simulink model "structuri_avansate"  (R2024a)
settings: Solver=VariableStepAuto  StartTime=0.0  StopTime=1000  RelTol=1e-3
values from neighbouring files (symbols this model uses):
  C = 9    [Proiect.m]
  h0 = 16.78    [Proiect.m]
  h1 = 19.66    [Proiect.m]
  k = 0.035    [Proiect.m]
  k11 = k2*k2+4*(k-k3)*k1    (= 0.0890826)    [Proiect.m]
  k12 = 8*(k-k3)    (= 0.2848)    [Proiect.m]
  k13 = 2*(k-k3)    (= 0.0712)    [Proiect.m]
  k2 = -0.015    [Proiect.m]
  kcompensare = (delta_h/(q1-q0))/(delta_h/delta_ua)    (= 0.16393442623)    [Proiect.m]
  kp = (delta_h/3)/delta_ua    (= 1.92)    [Proiect.m]
  q0 = 37.07    [Proiect.m]
undefined symbols (not defined in the file or in its folder): ki, ki1, ki2, kp1, kp2
libraries: slpidlib x6
(part 2 of 2)

== system structuri_avansate/ModelProces 3/Pompa/k11  ==
  k : Inport
  Add : Sum
  Constant : Constant  Value=4
  Product : Product
  Product1 : Product  Inputs=3
  Subtract : Sum  Inputs=+-
  k1 : Constant  Value=0.624
  k2 : Constant  Value=-0.015
  k3 : Constant  Value=-0.0006
  k11 : Outport
  wires:
  k2/1 -> Product/2, Product/1
  k/1 -> Subtract/1
  k3/1 -> Subtract/2
  Subtract/1 -> Product1/1
  k1/1 -> Product1/2
  Constant/1 -> Product1/3
  Product1/1 -> Add/1
  Product/1 -> Add/2
  Add/1 -> k11/1

== system structuri_avansate/ModelProces 3/Pompa/k12 ==
  k : Inport
  Product1 : Product
  Subtract : Sum  Inputs=+-
  "constant " : Constant  Value=8
  k3 : Constant  Value=-0.0006
  k12 : Outport
  wires:
  k/1 -> Subtract/1
  k3/1 -> Subtract/2
  Subtract/1 -> Product1/1
  "constant "/1 -> Product1/2
  Product1/1 -> k12/1

== system structuri_avansate/ModelProces 3/Pompa/k13 ==
  k : Inport
  Product1 : Product
  Subtract : Sum  Inputs=+-
  "constant " : Constant  Value=2
  k3 : Constant  Value=-0.0006
  k13 : Outport
  wires:
  k/1 -> Subtract/1
  k3/1 -> Subtract/2
  Subtract/1 -> Product1/1
  "constant "/1 -> Product1/2
  Product1/1 -> k13/1

== system structuri_avansate/ModelProces 4/Pompa/k11  ==
  k : Inport
  Add : Sum
  Constant : Constant  Value=4
  Product : Product
  Product1 : Product  Inputs=3
  Subtract : Sum  Inputs=+-
  k1 : Constant  Value=0.624
  k2 : Constant  Value=-0.015
  k3 : Constant  Value=-0.0006
  k11 : Outport
  wires:
  k2/1 -> Product/2, Product/1
  k/1 -> Subtract/1
  k3/1 -> Subtract/2
  Subtract/1 -> Product1/1
  k1/1 -> Product1/2
  Constant/1 -> Product1/3
  Product1/1 -> Add/1
  Product/1 -> Add/2
  Add/1 -> k11/1

== system structuri_avansate/ModelProces 4/Pompa/k12 ==
  k : Inport
  Product1 : Product
  Subtract : Sum  Inputs=+-
  "constant " : Constant  Value=8
  k3 : Constant  Value=-0.0006
  k12 : Outport
  wires:
  k/1 -> Subtract/1
  k3/1 -> Subtract/2
  Subtract/1 -> Product1/1
  "constant "/1 -> Product1/2
  Product1/1 -> k12/1

== system structuri_avansate/ModelProces 4/Pompa/k13 ==
  k : Inport
  Product1 : Product
  Subtract : Sum  Inputs=+-
  "constant " : Constant  Value=2
  k3 : Constant  Value=-0.0006
  k13 : Outport
  wires:
  k/1 -> Subtract/1
  k3/1 -> Subtract/2
  Subtract/1 -> Product1/1
  "constant "/1 -> Product1/2
  Product1/1 -> k13/1
